simulink model "DistillationColumn_MPC_R2020a"  (R2020a)
settings: Solver=ode23s  StartTime=0.0  StopTime=1e4  RelTol=1e-3
settings Model: Creator=tmlouw  LastModifiedBy=tmlouw
settings DebuggingCC: UnconnectedInputMsg=none  UnconnectedOutputMsg=none  UnconnectedLineMsg=none
settings ModelReferenceCC: EnableRefExpFcnMdlSchedulingChecks=off
settings RTWCC: Description=Generic Real-Time Target

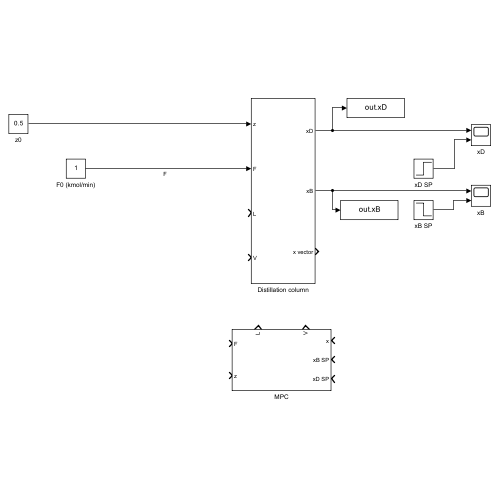
[thumbnail: Simulink's stored preview of the top-level diagram]
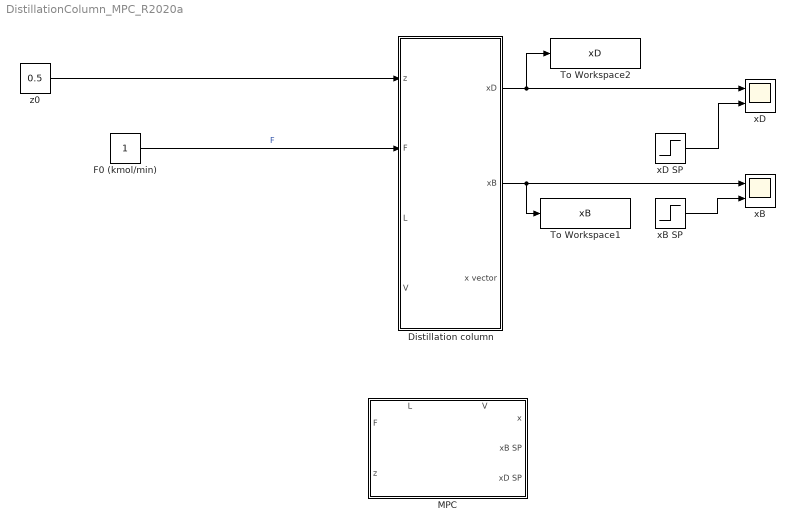
== system DistillationColumn_MPC_R2020a ==
  Distillation column : Subsystem
  F0 (kmol/min) : Constant
  MPC : Subsystem
      settings: PortSchema="{\"entries\":[{\"content\":{\"sides\":[{\"content\":{\"connectorIds\":[\"In1\",\"In2\",\"In3\"]},\"type\":\"ConnectorPlacement.EquallySpacedRectSide\",\"uuid\":\"fdb93da0-16e2-40e4-a743-261e7945158f\"},{\"content\":{\"connectorIds\":[\"In4\",\"In5\"],\"side\":\"RIGHT\"},\"type\":\"ConnectorPlacement.EquallySpacedRectSide\",\"uuid\":\"3cf89b73-5a07-47fa-8707-199400091fad\"},{\"content\":{\"connectorIds\":[\"Out1\",\"Out2\"],\"side\":\"TOP\"},\"type\":\"ConnectorPlacement.EquallySpacedRectSide\",\"uuid\":\"ff7b3035-6a5c-4512-8585-b641f6ec86e9\"}]},\"type\":\"ConnectorPlacement.EquallySpacedConnector\",\"uuid\":\"a06dce2d-e4e0-4b50-b4b6-566d92ea28b1\"}],\"packageUris\":[\"http://schema.mathworks.com/mf0/Connector/R2020b\"],\"version\":\"1.0\"}"
  To Workspace1 : ToWorkspace  VariableName=xB  SampleTime=10
      settings: Save2DSignal=2-D array (concatenate along first dimension)
  To Workspace2 : ToWorkspace  VariableName=xD  SampleTime=10
      settings: Save2DSignal=2-D array (concatenate along first dimension)
  xB : Scope  NumInputPorts=2
  xB SP : Step  Time=2500  Before=0.036  After=0.03  SampleTime=0
  xD : Scope  NumInputPorts=2
  xD SP : Step  Time=7500  Before=0.96  After=0.97  SampleTime=0
  z0 : Constant  Value=0.5
  wires:
  z0/1 -> Distillation column/1(z)
  F0 (kmol/min)/1 -> Distillation column/2(F)  "F"
  xD SP/1 -> xD/2
  xB SP/1 -> xB/2
  Distillation column/2(xB) -> xB/1, To Workspace1/1
  Distillation column/1(xD) -> xD/1, To Workspace2/1

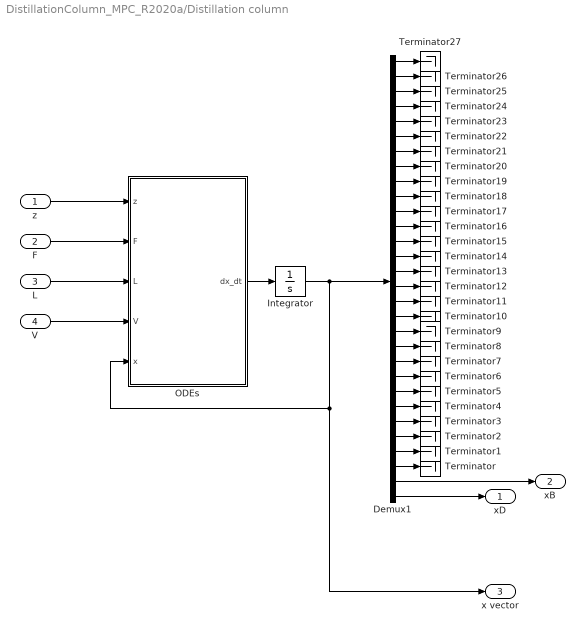
== system DistillationColumn_MPC_R2020a/Distillation column ==
  z : Inport
  F : Inport  Port=2
  L : Inport  Port=3
  V : Inport  Port=4
  Demux1 : Demux  Outputs=30
  Integrator : Integrator  InitialCondition=[linspace(0,0.99,28)'; 0.036; 0.96]  UpperSaturationLimit=1  LowerSaturationLimit=0
  ODEs : MATLAB Function  TreatAsAtomicUnit=on
  Terminator{,1..27} (28 alike) : Terminator
  xD : Outport
  xB : Outport  Port=2
  x vector : Outport  Port=3
  wires:
  F/1 -> ODEs/2(F)
  V/1 -> ODEs/4(V)
  ODEs/1(dx_dt) -> Integrator/1
  Demux1/29 -> xB/1
  L/1 -> ODEs/3(L)
  Demux1/30 -> xD/1
  z/1 -> ODEs/1(z)
  Demux1/20 -> Terminator8/1
  Demux1/16 -> Terminator12/1
  Demux1/14 -> Terminator14/1
  Demux1/17 -> Terminator11/1
  Demux1/23 -> Terminator5/1
  Demux1/9 -> Terminator19/1
  Demux1/8 -> Terminator20/1
  Demux1/11 -> Terminator17/1
  Demux1/12 -> Terminator16/1
  Demux1/27 -> Terminator1/1
  Demux1/1 -> Terminator27/1
  Demux1/13 -> Terminator15/1
  Demux1/6 -> Terminator22/1
  Integrator/1 -> x vector/1, ODEs/5(x), Demux1/1
  Demux1/4 -> Terminator24/1
  Demux1/19 -> Terminator9/1
  Demux1/24 -> Terminator4/1
  Demux1/25 -> Terminator3/1
  Demux1/5 -> Terminator23/1
  Demux1/18 -> Terminator10/1
  Demux1/2 -> Terminator26/1
  Demux1/28 -> Terminator/1
  Demux1/10 -> Terminator18/1
  Demux1/7 -> Terminator21/1
  Demux1/26 -> Terminator2/1
  Demux1/21 -> Terminator7/1
  Demux1/15 -> Terminator13/1
  Demux1/22 -> Terminator6/1
  Demux1/3 -> Terminator25/1

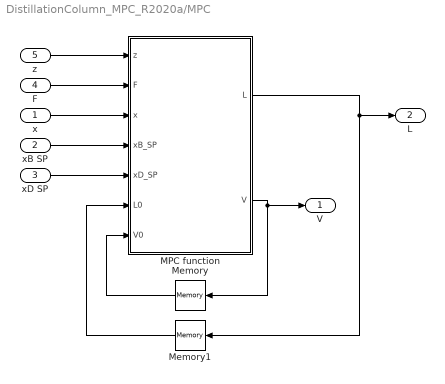
== system DistillationColumn_MPC_R2020a/MPC ==
  x : Inport
  xB SP : Inport  Port=2
  xD SP : Inport  Port=3
  F : Inport  Port=4
  z : Inport  Port=5
  MPC function : MATLAB Function  TreatAsAtomicUnit=on
  Memory : Memory  InitialCondition=0.6
  Memory1 : Memory  InitialCondition=1.1
  V : Outport
  L : Outport  Port=2
  wires:
  MPC function/1(L) -> Memory1/1, L/1
  MPC function/2(V) -> Memory/1, V/1
  F/1 -> MPC function/2(F)
  xB SP/1 -> MPC function/4(xB_SP)
  x/1 -> MPC function/3(x)
  xD SP/1 -> MPC function/5(xD_SP)
  z/1 -> MPC function/1(z)
  Memory1/1 -> MPC function/6(L0)
  Memory/1 -> MPC function/7(V0)

== matlab function DistillationColumn_MPC_R2020a/MPC/MPC function ==
  settings: updateMethod=DISCRETE  sampleTime=10
  data: z input; F input; x input; L output size=1; V output size=1; xB_SP input; xD_SP input; L0 input; V0 input
function [L, V] = MPC(z, F, x, xB_SP, xD_SP, L0, V0)
% Function representing an idealised MPC for the distillation column.
% Optimisation is performed over the reflux rate and the distillate flowrate as
% the distillate flowrate is clearly bounded between 0 and the feed flowrate F
%
% Inputs are defined as follows:
%   z: ~, feed composition
%   F: kmol/min, feed flowrate
%   x: ~, distillation column compositions
%   xB: ~, bottoms composition set-poit
%   xD: ~, distillate composition set-poit
%   L0: kmol/min, nominal reflux flowrate
%   V0: kmol/min, nominal vapour flowrate
%
% The calculated outputs are:
%   L: kmol/min, optimal reflux flowrate
%   V: kmol/min, optimal vapour flowrate

    dt = 10;  % min, MPC time step. Note this value needs to be changed in the function properties as well
    Nc = 2;   % ~, MPC control horizon
    Np = 5;   % ~, MPC prediction horizon
    opts = optimoptions('lsqnonlin','Algorithm','levenberg-marquardt'); % Optimisation algorithm
    
    % Initial guess for L and D over control horizon 
    L_guess = L0*ones(1, Nc);
    D_guess = (V0 - L0)*ones(1, Nc);
    u0 = [L_guess, D_guess];
    
    % Upper and lower bounds on L and D
    lb = zeros(1, 2*Nc); % Lower bounds for L and D are both zero
    ub = [inf*ones(1, Nc), F*ones(1,Nc)];     % No upper bound on L, but D may not exceed F
    
    % Determine optimal L and D
    u_opt = lsqnonlin(@(u) objectiveFunction(u, z, F, x, xB_SP, xD_SP, L0, V0, Nc, Np, dt), u0, lb, ub, opts);
    L = u_opt(1);
    D = u_opt(Nc+1);
    V = L+D; % Calculate optimal V from L and D
end

function R = objectiveFunction(u, z, F, x0, xB_SP, xD_SP, L0, V0, Nc, Np,dt)
    % Define control horizon and create a function fL and fV which will
    % return L and V as functions of time, to be used in numerical integration
    t_control = -dt:dt:dt*(Nc-1);
    L = u(1:Nc);     
    D = u(Nc+1:end); 
    V = L+D;         
    fL = griddedInterpolant(t_control, [L0, L], 'previous');
    fV = griddedInterpolant(t_control, [V0, V], 'previous');

    % Define prediction horizon and predict system response given L and V
    t_predict = 0:dt:dt*Np;
    [~, x] = ode45(@(t, x) predictMPC(t, z, F, fL, fV, x), t_predict, x0);

    % Determine the bottoms- and distillate composition as a function of time
    xB = x(:,29);
    xD = x(:,30);

    % Return a vector of residuals "R", where the objective function to be minimized 
    % can be calculated using J = R'R (this is useful to speed up calculations)
    R = [(xB - xB_SP); (xD - xD_SP); 0.01*(L - [L0, L(1:end-1)])'; 0.01*(V - [V0, V(1:end-1)])'];

end

function dx_dt = predictMPC(t, z, F, fL, fV, x)
    % ODEs representing a 30-tray distillation column for benzene/toluene
    % separation. All molar hold-ups are constant, only composition varies.
    % The feed is assumed to be a saturated liquid.
    %
    % This function is silimar to "distillationColumn", used to simulate
    % the process itself, except the inputs L and V are provided as
    % functions of time.
    % Parameters may be changed to simulate plant-model mismatch.
    % Inputs are defined as follows:
    %
    %   t: min, time from start of prediction
    %   z: ~, feed composition
    %   F: kmol/min, feed flowrate
    %   fL: kmol/min, reflux flowrate as a function of time
    %   fV: kmol/min, vapour flowrate as a function of time
    % Input "x" has 30 elements
    %   x(1:28): ~, composition on stages 1-28
    %   x(29): ~, bottoms composition
    %   x(30): ~, condenser composition
    
    nB = 100;  % kmol, molar hold-up in reboiler
    n = 10;    % kmol, molar hold-up per tray
    nD = 100;  % kmol, molar hold-up in condenser
    
    N = 28; % ~, Number of stages
    f = 15; % ~, Feed stage
    
    xB = x(29); % ~, bottoms composition
    xD = x(30); % ~, distillate composition
    L = fL(t);  % kmol/min, reflux flowrate
    V = fV(t);  % kmol/min, vapour flowrate
    LB = L + F;    % kmol/min, liquid flowrate below feed tray
    B = L + F - V; % kmol/min, bottoms flowrate
    
    alpha = 2.5; % ~, relative volatility
    fy = @(x) alpha*x / (1 + (alpha-1)*x); % ~, vapour composition given specified liquid composition "x"
    
    % Calculate the vapour composition on each tray, as well as over the reboiler
    y = zeros(28,1);
    for i = 1:N
        y(i) = fy(x(i));
    end
    yB = fy(xB);
    
    % Create an empty array representing the derivative of composition wrt time
    dx_dt = zeros(30,1);
    
    % Calculate time rate of change of composition for the reboiler, each tray,
    % and the distillate, using a molar balance over each
    % Reboiler and first stage
    dxB_dt = ( LB*x(1) - B*xB - V*yB )/nB;
    dx_dt(1) = ( LB*(x(2) - x(1)) + V*(yB - y(1)) )/n;
    % Below feed
    for i = 2:f-1
        dx_dt(i) = ( LB*(x(i+1) - x(i)) + V*(y(i-1) - y(i)) )/n;
    end
    % Feed stage
    dx_dt(f) = ( F*z + L*x(f+1) - LB*x(f) + V*(y(f-1) - y(f)) )/n;
    % Above feed
    for i = f+1:N-1
        dx_dt(i) = ( L*(x(i+1) - x(i)) + V*(y(i-1) - y(i)) )/n;
    end
    % Top stage and condenser
    dx_dt(N) =  ( L*(xD - x(N)) + V*(y(N-1) - y(N)) )/n;
    dxD_dt = V*(y(N) - xD)/nD;
    
    dx_dt(29) = dxB_dt;
    dx_dt(30) = dxD_dt;
end

== matlab function DistillationColumn_MPC_R2020a/Distillation column/ODEs ==
  data: z input; dx_dt output; F input; L input; V input; x input
function dx_dt = distillationColumn(z, F, L, V, x)
% ODEs representing a 28-tray distillation column for benzene/toluene
% separation. All molar hold-ups are constant, only composition varies.
% The feed is assumed to be a saturated liquid.
%
% Inputs are defined as follows:
%   z: ~, feed composition
%   F: kmol/min, feed flowrate
%   L: kmol/min, reflux flowrate
%   V: kmol/min, vapour flowrate
% Input "x" has 30 elements
%   x(1:28): ~, composition on stages 1-28
%   x(29): ~, bottoms composition
%   x(30): ~, condenser composition

nB = 100;  % kmol, molar hold-up in reboiler
n = 10;    % kmol, molar hold-up per tray
nD = 100;  % kmol, molar hold-up in condenser

N = 28; % ~, Number of stages
f = 15; % ~, Feed stage

xB = x(29); % ~, bottoms composition
xD = x(30); % ~, distillate composition
LB = L + F;    % kmol/min, liquid flowrate below feed tray
B = L + F - V; % kmol/min, bottoms flowrate

alpha = 2.5; % ~, relative volatility
fy = @(x) alpha*x / (1 + (alpha-1)*x); % ~, vapour composition given specified liquid composition "x"

% Calculate the vapour composition on each tray, as well as over the reboiler
y = zeros(28,1);
for i = 1:N
    y(i) = fy(x(i));
end
yB = fy(xB);

% Create an empty array representing the derivative of composition wrt time
dx_dt = zeros(30,1);

% Calculate time rate of change of composition for the reboiler, each tray,
% and the distillate, using a molar balance over each
% Reboiler and first stage
dxB_dt = ( LB*x(1) - B*xB - V*yB )/nB;
dx_dt(1) = ( LB*(x(2) - x(1)) + V*(yB - y(1)) )/n;
% Below feed
for i = 2:f-1
    dx_dt(i) = ( LB*(x(i+1) - x(i)) + V*(y(i-1) - y(i)) )/n;
end
% Feed stage
dx_dt(f) = ( F*z + L*x(f+1) - LB*x(f) + V*(y(f-1) - y(f)) )/n;
% Above feed
for i = f+1:N-1
    dx_dt(i) = ( L*(x(i+1) - x(i)) + V*(y(i-1) - y(i)) )/n;
end
% Top stage and condenser
dx_dt(N) =  ( L*(xD - x(N)) + V*(y(N-1) - y(N)) )/n;
dxD_dt = V*(y(N) - xD)/nD;

dx_dt(29) = dxB_dt;
dx_dt(30) = dxD_dt;
